simulink model "RocketPlant-org"  (R2025b)
settings: Solver=VariableStepAuto  StartTime=0.0  StopTime=10.0  RelTol=1e-3
undefined symbols (not defined in the file): fluid
libraries: metux_library x9
settings Model: DataDictionary=motorData.sldd  Creator=karadeli  LastModifiedBy=karadeli

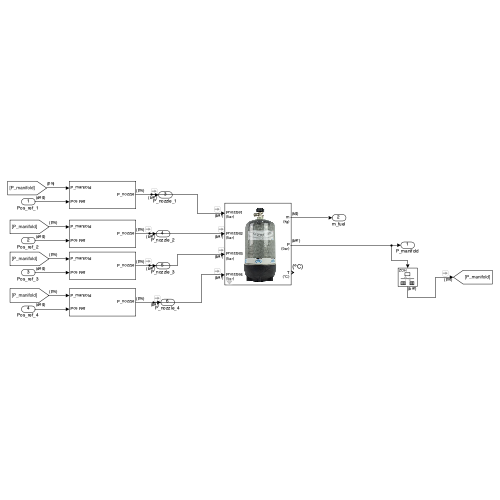
[thumbnail: Simulink's stored preview of the top-level diagram]
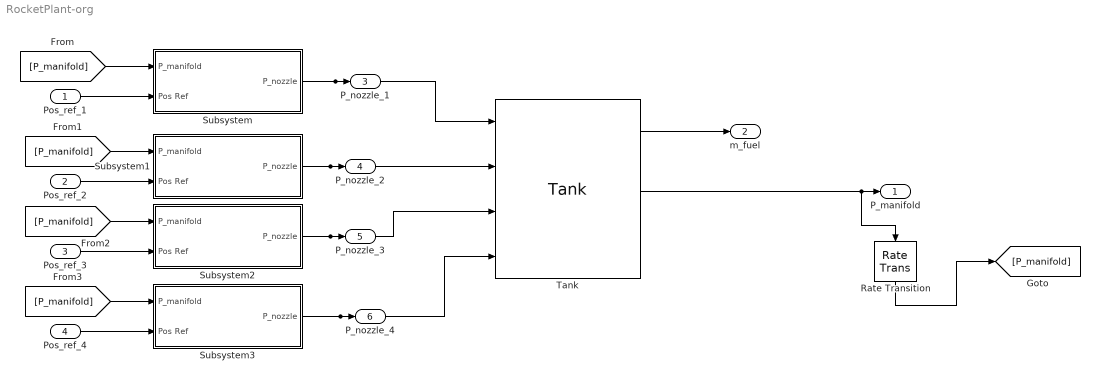
== system RocketPlant-org ==
  Pos_ref_1 : Inport  Unit=deg
  Pos_ref_2 : Inport  Port=2  Unit=deg
  Pos_ref_3 : Inport  Port=3  Unit=deg
  Pos_ref_4 : Inport  Port=4  Unit=deg
  Rate Transition : RateTransition  OutPortSampleTime=1/1000
  Subsystem : Subsystem
  Subsystem1 : Subsystem
  Subsystem2 : Subsystem
  Subsystem3 : Subsystem
  Tank : metux_library/Tank  P0=300  T0=25  mdotGain=fluid.mdotGain  V=fluid.V  R=fluid.R  Cv=fluid.Cv  Patm=fluid.Patm
  P_manifold : Outport
  m_fuel : Outport  Port=2
  P_nozzle_1 : Outport  Port=3  Unit=bar
  P_nozzle_2 : Outport  Port=4  Unit=bar
  P_nozzle_3 : Outport  Port=5  Unit=bar
  P_nozzle_4 : Outport  Port=6  Unit=bar
  wires:
  [P_manifold] -> Subsystem/1(P_manifold)
  Pos_ref_1/1 -> Subsystem/2(Pos Ref)
  Subsystem/1(P_nozzle) -> Tank/1, P_nozzle_1/1
  Subsystem1/1(P_nozzle) -> P_nozzle_2/1, Tank/2
  Subsystem2/1(P_nozzle) -> P_nozzle_3/1, Tank/3
  Subsystem3/1(P_nozzle) -> P_nozzle_4/1, Tank/4
  [P_manifold] -> Subsystem1/1(P_manifold)
  Pos_ref_2/1 -> Subsystem1/2(Pos Ref)
  Pos_ref_4/1 -> Subsystem3/2(Pos Ref)
  Pos_ref_3/1 -> Subsystem2/2(Pos Ref)
  [P_manifold] -> Subsystem3/1(P_manifold)
  [P_manifold] -> Subsystem2/1(P_manifold)
  Tank/1 -> m_fuel/1
  Rate Transition/1 -> [P_manifold]
  Tank/2 -> P_manifold/1, Rate Transition/1

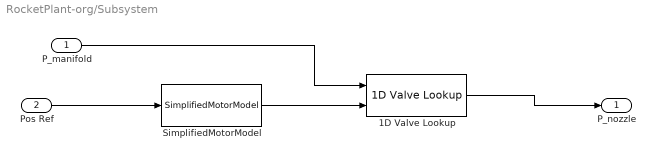
== system RocketPlant-org/Subsystem ==
  P_manifold : Inport
  Pos Ref : Inport  Port=2
  1D Valve Lookup : metux_library/1D Valve Lookup  SystemSampleTime=-1  VariantActivationTime=update diagram  EmptyChoice=off  PassThrough=off  PassThroughVariantControl=(default)  EmptyChoiceVariantControl=(default)  AllowFlexibleInterface=on  Latency=0  AutoFrameSizeCalculation=off
  SimplifiedMotorModel : metux_library/SimplifiedMotorModel  SystemSampleTime=-1  VariantActivationTime=update diagram  EmptyChoice=off  PassThrough=off  PassThroughVariantControl=(default)  EmptyChoiceVariantControl=(default)  AllowFlexibleInterface=on  Latency=0  AutoFrameSizeCalculation=off
  P_nozzle : Outport
  wires:
  Pos Ref/1 -> SimplifiedMotorModel/1
  P_manifold/1 -> 1D Valve Lookup/1
  1D Valve Lookup/1 -> P_nozzle/1
  SimplifiedMotorModel/1 -> 1D Valve Lookup/2

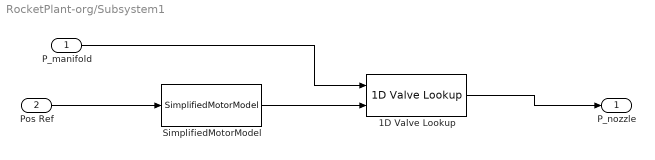
== system RocketPlant-org/Subsystem1 ==
  P_manifold : Inport
  Pos Ref : Inport  Port=2
  1D Valve Lookup : metux_library/1D Valve Lookup  SystemSampleTime=-1  VariantActivationTime=update diagram  EmptyChoice=off  PassThrough=off  PassThroughVariantControl=(default)  EmptyChoiceVariantControl=(default)  AllowFlexibleInterface=on  Latency=0  AutoFrameSizeCalculation=off
  SimplifiedMotorModel : metux_library/SimplifiedMotorModel  SystemSampleTime=-1  VariantActivationTime=update diagram  EmptyChoice=off  PassThrough=off  PassThroughVariantControl=(default)  EmptyChoiceVariantControl=(default)  AllowFlexibleInterface=on  Latency=0  AutoFrameSizeCalculation=off
  P_nozzle : Outport
  wires:
  SimplifiedMotorModel/1 -> 1D Valve Lookup/2
  1D Valve Lookup/1 -> P_nozzle/1
  P_manifold/1 -> 1D Valve Lookup/1
  Pos Ref/1 -> SimplifiedMotorModel/1

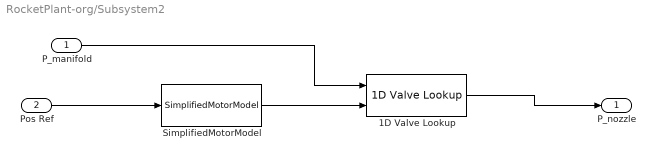
== system RocketPlant-org/Subsystem2 ==
  P_manifold : Inport
  Pos Ref : Inport  Port=2
  1D Valve Lookup : metux_library/1D Valve Lookup  SystemSampleTime=-1  VariantActivationTime=update diagram  EmptyChoice=off  PassThrough=off  PassThroughVariantControl=(default)  EmptyChoiceVariantControl=(default)  AllowFlexibleInterface=on  Latency=0  AutoFrameSizeCalculation=off
  SimplifiedMotorModel : metux_library/SimplifiedMotorModel  SystemSampleTime=-1  VariantActivationTime=update diagram  EmptyChoice=off  PassThrough=off  PassThroughVariantControl=(default)  EmptyChoiceVariantControl=(default)  AllowFlexibleInterface=on  Latency=0  AutoFrameSizeCalculation=off
  P_nozzle : Outport
  wires:
  Pos Ref/1 -> SimplifiedMotorModel/1
  P_manifold/1 -> 1D Valve Lookup/1
  1D Valve Lookup/1 -> P_nozzle/1
  SimplifiedMotorModel/1 -> 1D Valve Lookup/2

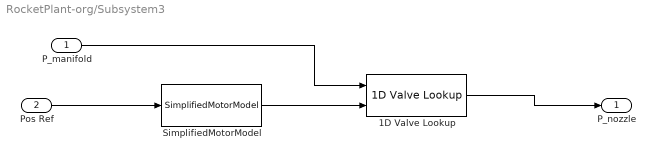
== system RocketPlant-org/Subsystem3 ==
  P_manifold : Inport
  Pos Ref : Inport  Port=2
  1D Valve Lookup : metux_library/1D Valve Lookup  SystemSampleTime=-1  VariantActivationTime=update diagram  EmptyChoice=off  PassThrough=off  PassThroughVariantControl=(default)  EmptyChoiceVariantControl=(default)  AllowFlexibleInterface=on  Latency=0  AutoFrameSizeCalculation=off
  SimplifiedMotorModel : metux_library/SimplifiedMotorModel  SystemSampleTime=-1  VariantActivationTime=update diagram  EmptyChoice=off  PassThrough=off  PassThroughVariantControl=(default)  EmptyChoiceVariantControl=(default)  AllowFlexibleInterface=on  Latency=0  AutoFrameSizeCalculation=off
  P_nozzle : Outport
  wires:
  SimplifiedMotorModel/1 -> 1D Valve Lookup/2
  1D Valve Lookup/1 -> P_nozzle/1
  P_manifold/1 -> 1D Valve Lookup/1
  Pos Ref/1 -> SimplifiedMotorModel/1
